simulink library "halout"  (R2021b)
settings: Solver=VariableStepAuto  StartTime=0.0  StopTime=10.0  RelTol=1e-3
undefined symbols (not defined in the file): C_TASK_5MS_S, FALSE, KHAL_CAN1FD1APS3E2E_flg, KHAL_CAN1FD1APS3TxReq_flg, KHAL_CAN1FD1VCU2E2E_flg, KHAL_CAN1FD1VCU2TxReq_flg, KHAL_CAN1FD1VCU3E2E_flg, KHAL_CAN1FD1VCU3TxReq_flg, KHAL_CAN1TxReq_flg, KHAL_CAN1VMCFCM1E2E_flg, KHAL_CAN1VMCFCM1TxReq_flg, KHAL_CAN2TxReq_flg, KHAL_CAN3FD3VCU1toNIDECTxReq_flg, KHAL_CAN3FD3VCU1TxReq_flg, KHAL_CAN3FD3VCU2E2E_flg, KHAL_CAN3FD3VCU2toNIDECE2E_flg, KHAL_CAN3FD3VCU2toNIDECTxReq_flg, KHAL_CAN3FD3VCU2TxReq_flg, KHAL_CAN3TxReq_flg, KHAL_CAN4FD4CE1000E2E_flg, KHAL_CAN4FD4CE1000TxReq_flg, KHAL_CAN4TxReq_flg, KHAL_CAN5TxReq_flg, KHAL_CAN6FD6APS3E2E_flg, KHAL_CAN6FD6APS3TxReq_flg, KHAL_CAN6FD6VCU2E2E_flg, KHAL_CAN6FD6VCU2TxReq_flg, KHAL_CAN6TxReq_flg, ONE_INT, TRUE, ZERO_INT
libraries: FVT_lib x551, simulink x244
(part 16 of 26)

== system halout/HAL_OUT/CAN1/FD1_VCU3_0x159/RrEDURealDrvOrBRgnTq ==
  RrEDURealDrvOrBRgnTq : Inport
  Data Type Conversion : DataTypeConversion  OutDataTypeStr=uint16  RndMeth=Round
  convert_out : FVT_lib/hal/convert_out  gain=0.5  offset=-5300
  CAN1_Rr_EDURealDrvOrBRgnTq : Outport
  wires:
  Data Type Conversion/1 -> CAN1_Rr_EDURealDrvOrBRgnTq/1
  convert_out/1 -> Data Type Conversion/1
  RrEDURealDrvOrBRgnTq/1 -> convert_out/1

== system halout/HAL_OUT/CAN1/FD1_VCU3_0x159/RrEDUSpd ==
  RrEDUSpd : Inport
  Data Type Conversion : DataTypeConversion  OutDataTypeStr=uint16  RndMeth=Round
  convert_out : FVT_lib/hal/convert_out  gain=1  offset=-2000
  CAN1_Rr_EDUSpd : Outport
  wires:
  Data Type Conversion/1 -> CAN1_Rr_EDUSpd/1
  convert_out/1 -> Data Type Conversion/1
  RrEDUSpd/1 -> convert_out/1

== system halout/HAL_OUT/CAN1/FD1_VCU3_0x159/RrEDUSpdValid ==
  RrEDUSpdValid : Inport
  Data Type Conversion : DataTypeConversion  OutDataTypeStr=uint8  RndMeth=Round
  CAN1_Rr_EDUSpdValid : Outport
  wires:
  Data Type Conversion/1 -> CAN1_Rr_EDUSpdValid/1
  RrEDUSpdValid/1 -> Data Type Conversion/1

== system halout/HAL_OUT/CAN1/FD1_VCU3_0x159/RrRgnDecrSta ==
  RrRgnDecrSta : Inport
  Data Type Conversion : DataTypeConversion  OutDataTypeStr=uint8  RndMeth=Round
  CAN1_Rr_RgnDecrSta : Outport
  wires:
  Data Type Conversion/1 -> CAN1_Rr_RgnDecrSta/1
  RrRgnDecrSta/1 -> Data Type Conversion/1

== system halout/HAL_OUT/CAN1/FD1_VCU3_0x159/RrRgnPermSta ==
  RrRgnPermSta : Inport
  Data Type Conversion : DataTypeConversion  OutDataTypeStr=uint8  RndMeth=Round
  CAN1_Rr_RgnPermSta : Outport
  wires:
  Data Type Conversion/1 -> CAN1_Rr_RgnPermSta/1
  RrRgnPermSta/1 -> Data Type Conversion/1

== system halout/HAL_OUT/CAN1/FD1_VMC1_0x17F/AccCalcuPID ==
  AccCalcuPID : Inport
  Data Type Conversion : DataTypeConversion  OutDataTypeStr=uint16  RndMeth=Round
  convert_out : FVT_lib/hal/convert_out  gain=0.05  offset=-15
  CAN1_AccCalcuPID : Outport
  wires:
  Data Type Conversion/1 -> CAN1_AccCalcuPID/1
  convert_out/1 -> Data Type Conversion/1
  AccCalcuPID/1 -> convert_out/1

== system halout/HAL_OUT/CAN1/FD1_VMC1_0x17F/CCMSASpdWar ==
  CCMSASpdWar : Inport
  Data Type Conversion : DataTypeConversion  OutDataTypeStr=uint8  RndMeth=Round
  CAN1_CCMSA_SpdWar : Outport
  wires:
  Data Type Conversion/1 -> CAN1_CCMSA_SpdWar/1
  CCMSASpdWar/1 -> Data Type Conversion/1

== system halout/HAL_OUT/CAN1/FD1_VMC1_0x17F/DISCButtSta ==
  DISCButtSta : Inport
  Data Type Conversion : DataTypeConversion  OutDataTypeStr=uint8  RndMeth=Round
  CAN1_DISC_ButtSta : Outport
  wires:
  Data Type Conversion/1 -> CAN1_DISC_ButtSta/1
  DISCButtSta/1 -> Data Type Conversion/1

== system halout/HAL_OUT/CAN1/FD1_VMC1_0x17F/DISCDISCTargetSpd ==
  DISCDISCTargetSpd : Inport
  Data Type Conversion : DataTypeConversion  OutDataTypeStr=uint16  RndMeth=Round
  convert_out : FVT_lib/hal/convert_out  gain=0.125  offset=0
  CAN1_DISC_DISCTargetSpd : Outport
  wires:
  Data Type Conversion/1 -> CAN1_DISC_DISCTargetSpd/1
  convert_out/1 -> Data Type Conversion/1
  DISCDISCTargetSpd/1 -> convert_out/1

== system halout/HAL_OUT/CAN1/FD1_VMC1_0x17F/DISCDISCTurn ==
  DISCDISCTurn : Inport
  Data Type Conversion : DataTypeConversion  OutDataTypeStr=uint8  RndMeth=Round
  CAN1_DISC_DISCTurn : Outport
  wires:
  Data Type Conversion/1 -> CAN1_DISC_DISCTurn/1
  DISCDISCTurn/1 -> Data Type Conversion/1

== system halout/HAL_OUT/CAN1/FD1_VMC1_0x17F/DISCReqAcc ==
  DISCReqAcc : Inport
  Data Type Conversion : DataTypeConversion  OutDataTypeStr=uint16  RndMeth=Round
  convert_out : FVT_lib/hal/convert_out  gain=0.05  offset=-15
  CAN1_DISCReqAcc : Outport
  wires:
  Data Type Conversion/1 -> CAN1_DISCReqAcc/1
  convert_out/1 -> Data Type Conversion/1
  DISCReqAcc/1 -> convert_out/1

== system halout/HAL_OUT/CAN1/FD1_VMC1_0x17F/DISCSta ==
  DISCSta : Inport
  Data Type Conversion : DataTypeConversion  OutDataTypeStr=uint8  RndMeth=Round
  CAN1_DISC_Sta : Outport
  wires:
  Data Type Conversion/1 -> CAN1_DISC_Sta/1
  DISCSta/1 -> Data Type Conversion/1

== system halout/HAL_OUT/CAN1/FD1_VMC1_0x17F/FeatArbitrFinal ==
  FeatArbitrFinal : Inport
  Data Type Conversion : DataTypeConversion  OutDataTypeStr=uint8  RndMeth=Round
  CAN1_FeatArbitrFinal : Outport
  wires:
  Data Type Conversion/1 -> CAN1_FeatArbitrFinal/1
  FeatArbitrFinal/1 -> Data Type Conversion/1

== system halout/HAL_OUT/CAN1/FD1_VMC1_0x17F/FeatArbitrSta ==
  FeatArbitrSta : Inport
  Data Type Conversion : DataTypeConversion  OutDataTypeStr=uint8  RndMeth=Round
  CAN1_FeatArbitrSta : Outport
  wires:
  Data Type Conversion/1 -> CAN1_FeatArbitrSta/1
  FeatArbitrSta/1 -> Data Type Conversion/1

== system halout/HAL_OUT/CAN1/FD1_VMC1_0x17F/FeatReqSpd ==
  FeatReqSpd : Inport
  Data Type Conversion : DataTypeConversion  OutDataTypeStr=uint16  RndMeth=Round
  convert_out : FVT_lib/hal/convert_out  gain=0.125  offset=0
  CAN1_FeatReqSpd : Outport
  wires:
  Data Type Conversion/1 -> CAN1_FeatReqSpd/1
  convert_out/1 -> Data Type Conversion/1
  FeatReqSpd/1 -> convert_out/1

== system halout/HAL_OUT/CAN1/FD1_VMC1_0x17F/FeatSetSpdFinalraw32 ==
  FeatSetSpdFinalraw32 : Inport
  Data Type Conversion : DataTypeConversion  OutDataTypeStr=uint8  RndMeth=Round
  CAN1_FeatSetSpdFinal_raw32 : Outport
  wires:
  Data Type Conversion/1 -> CAN1_FeatSetSpdFinal_raw32/1
  FeatSetSpdFinalraw32/1 -> Data Type Conversion/1

== system halout/HAL_OUT/CAN1/FD1_VMC1_0x17F/FrontRearSlipRatioCtrl ==
  FrontRearSlipRatioCtrl : Inport
  Data Type Conversion : DataTypeConversion  OutDataTypeStr=uint8  RndMeth=Round
  CAN1_FrontRearSlipRatioCtrl : Outport
  wires:
  Data Type Conversion/1 -> CAN1_FrontRearSlipRatioCtrl/1
  FrontRearSlipRatioCtrl/1 -> Data Type Conversion/1

== system halout/HAL_OUT/CAN1/FD1_VMC1_0x17F/JerkPCT ==
  JerkPCT : Inport
  Data Type Conversion : DataTypeConversion  OutDataTypeStr=uint8  RndMeth=Round
  CAN1_JerkPCT : Outport
  wires:
  Data Type Conversion/1 -> CAN1_JerkPCT/1
  JerkPCT/1 -> Data Type Conversion/1

== system halout/HAL_OUT/CAN1/FD1_VMC1_0x17F/LatAccCtrl ==
  LatAccCtrl : Inport
  Data Type Conversion : DataTypeConversion  OutDataTypeStr=uint8  RndMeth=Round
  CAN1_LatAccCtrl : Outport
  wires:
  Data Type Conversion/1 -> CAN1_LatAccCtrl/1
  LatAccCtrl/1 -> Data Type Conversion/1

== system halout/HAL_OUT/CAN1/FD1_VMC1_0x17F/LateralCtrl ==
  LateralCtrl : Inport
  Data Type Conversion : DataTypeConversion  OutDataTypeStr=uint8  RndMeth=Round
  CAN1_LateralCtrl : Outport
  wires:
  Data Type Conversion/1 -> CAN1_LateralCtrl/1
  LateralCtrl/1 -> Data Type Conversion/1

== system halout/HAL_OUT/CAN1/FD1_VMC1_0x17F/LimitPCT ==
  LimitPCT : Inport
  Data Type Conversion : DataTypeConversion  OutDataTypeStr=uint8  RndMeth=Round
  CAN1_LimitPCT : Outport
  wires:
  Data Type Conversion/1 -> CAN1_LimitPCT/1
  LimitPCT/1 -> Data Type Conversion/1

== system halout/HAL_OUT/CAN1/FD1_VMC1_0x17F/MeterIndSpeedraw32 ==
  MeterIndSpeedraw32 : Inport
  Data Type Conversion : DataTypeConversion  OutDataTypeStr=uint8  RndMeth=Round
  CAN1_MeterIndSpeed_raw32 : Outport
  wires:
  Data Type Conversion/1 -> CAN1_MeterIndSpeed_raw32/1
  MeterIndSpeedraw32/1 -> Data Type Conversion/1

== system halout/HAL_OUT/CAN1/FD1_VMC1_0x17F/RearWhlSlipRatioCtrl ==
  RearWhlSlipRatioCtrl : Inport
  Data Type Conversion : DataTypeConversion  OutDataTypeStr=uint8  RndMeth=Round
  CAN1_RearWhlSlipRatioCtrl : Outport
  wires:
  Data Type Conversion/1 -> CAN1_RearWhlSlipRatioCtrl/1
  RearWhlSlipRatioCtrl/1 -> Data Type Conversion/1

== system halout/HAL_OUT/CAN1/FD1_VMC1_0x17F/SPD2ACCAct ==
  SPD2ACCAct : Inport
  Data Type Conversion : DataTypeConversion  OutDataTypeStr=uint8  RndMeth=Round
  CAN1_SPD2ACCAct : Outport
  wires:
  Data Type Conversion/1 -> CAN1_SPD2ACCAct/1
  SPD2ACCAct/1 -> Data Type Conversion/1

== system halout/HAL_OUT/CAN1/FD1_VMC1_0x17F/SafetyCtrl ==
  SafetyCtrl : Inport
  Data Type Conversion : DataTypeConversion  OutDataTypeStr=uint8  RndMeth=Round
  CAN1_SafetyCtrl : Outport
  wires:
  Data Type Conversion/1 -> CAN1_SafetyCtrl/1
  SafetyCtrl/1 -> Data Type Conversion/1

== system halout/HAL_OUT/CAN1/FD1_VMC1_0x17F/SingleWhlSlipRatioCtrl ==
  SingleWhlSlipRatioCtrl : Inport
  Data Type Conversion : DataTypeConversion  OutDataTypeStr=uint8  RndMeth=Round
  CAN1_SingleWhlSlipRatioCtrl : Outport
  wires:
  Data Type Conversion/1 -> CAN1_SingleWhlSlipRatioCtrl/1
  SingleWhlSlipRatioCtrl/1 -> Data Type Conversion/1

== system halout/HAL_OUT/CAN1/FD1_VMC1_0x17F/TimeGapCalcu ==
  TimeGapCalcu : Inport
  Data Type Conversion : DataTypeConversion  OutDataTypeStr=uint8  RndMeth=Round
  convert_out : FVT_lib/hal/convert_out  gain=0.1  offset=0
  CAN1_TimeGapCalcu : Outport
  wires:
  Data Type Conversion/1 -> CAN1_TimeGapCalcu/1
  convert_out/1 -> Data Type Conversion/1
  TimeGapCalcu/1 -> convert_out/1

== system halout/HAL_OUT/CAN1/FD1_VMC1_0x17F/VMCACCCtrlAvail ==
  VMCACCCtrlAvail : Inport
  Data Type Conversion : DataTypeConversion  OutDataTypeStr=uint8  RndMeth=Round
  CAN1_VMC_ACCCtrlAvail : Outport
  wires:
  Data Type Conversion/1 -> CAN1_VMC_ACCCtrlAvail/1
  VMCACCCtrlAvail/1 -> Data Type Conversion/1

== system halout/HAL_OUT/CAN1/FD1_VMC1_0x17F/VMCAEBCtrlAvail ==
  VMCAEBCtrlAvail : Inport
  Data Type Conversion : DataTypeConversion  OutDataTypeStr=uint8  RndMeth=Round
  CAN1_VMC_AEBCtrlAvail : Outport
  wires:
  Data Type Conversion/1 -> CAN1_VMC_AEBCtrlAvail/1
  VMCAEBCtrlAvail/1 -> Data Type Conversion/1

== system halout/HAL_OUT/CAN1/FD1_VMC1_0x17F/VMCCCCtrlAvail ==
  VMCCCCtrlAvail : Inport
  Data Type Conversion : DataTypeConversion  OutDataTypeStr=uint8  RndMeth=Round
  CAN1_VMC_CCCtrlAvail : Outport
  wires:
  Data Type Conversion/1 -> CAN1_VMC_CCCtrlAvail/1
  VMCCCCtrlAvail/1 -> Data Type Conversion/1

== system halout/HAL_OUT/CAN1/FD1_VMC1_0x17F/VMCMSACtrlAvail ==
  VMCMSACtrlAvail : Inport
  Data Type Conversion : DataTypeConversion  OutDataTypeStr=uint8  RndMeth=Round
  CAN1_VMC_MSACtrlAvail : Outport
  wires:
  Data Type Conversion/1 -> CAN1_VMC_MSACtrlAvail/1
  VMCMSACtrlAvail/1 -> Data Type Conversion/1

== system halout/HAL_OUT/CAN1/FD1_VMC1_0x17F/VMCVCUACCCtrlAvail ==
  VMCVCUACCCtrlAvail : Inport
  Data Type Conversion : DataTypeConversion  OutDataTypeStr=uint8  RndMeth=Round
  CAN1_VMC_VCU_ACC_CtrlAvail : Outport
  wires:
  Data Type Conversion/1 -> CAN1_VMC_VCU_ACC_CtrlAvail/1
  VMCVCUACCCtrlAvail/1 -> Data Type Conversion/1

== system halout/HAL_OUT/CAN1/FD1_VMC1_0x17F/VMCVCUAPSCtrlAvailflg ==
  VMCVCUAPSCtrlAvailflg : Inport
  Data Type Conversion : DataTypeConversion  OutDataTypeStr=uint8  RndMeth=Round
  CAN1_VMC_VCU_APSCtrlAvail_flg : Outport
  wires:
  Data Type Conversion/1 -> CAN1_VMC_VCU_APSCtrlAvail_flg/1
  VMCVCUAPSCtrlAvailflg/1 -> Data Type Conversion/1

== system halout/HAL_OUT/CAN1/FD1_VMC1_0x17F/VMCVCUAccPedalOverride ==
  VMCVCUAccPedalOverride : Inport
  Data Type Conversion : DataTypeConversion  OutDataTypeStr=uint8  RndMeth=Round
  CAN1_VMC_VCU_AccPedal_Override : Outport
  wires:
  Data Type Conversion/1 -> CAN1_VMC_VCU_AccPedal_Override/1
  VMCVCUAccPedalOverride/1 -> Data Type Conversion/1

== system halout/HAL_OUT/CAN1/FD1_VMC1_0x17F/VMCVCUCCCrlSta ==
  VMCVCUCCCrlSta : Inport
  Data Type Conversion : DataTypeConversion  OutDataTypeStr=uint8  RndMeth=Round
  CAN1_VMC_VCU_CC_Crl_Sta : Outport
  wires:
  Data Type Conversion/1 -> CAN1_VMC_VCU_CC_Crl_Sta/1
  VMCVCUCCCrlSta/1 -> Data Type Conversion/1

== system halout/HAL_OUT/CAN1/FD1_VMC1_0x17F/VMCVCUMSACrlSta ==
  VMCVCUMSACrlSta : Inport
  Data Type Conversion : DataTypeConversion  OutDataTypeStr=uint8  RndMeth=Round
  CAN1_VMC_VCU_MSA_Crl_Sta : Outport
  wires:
  Data Type Conversion/1 -> CAN1_VMC_VCU_MSA_Crl_Sta/1
  VMCVCUMSACrlSta/1 -> Data Type Conversion/1

== system halout/HAL_OUT/CAN1/FD1_VMC1_0x17F/VehicleSpeedkph ==
  VehicleSpeedkph : Inport
  Data Type Conversion : DataTypeConversion  OutDataTypeStr=uint16  RndMeth=Round
  convert_out : FVT_lib/hal/convert_out  gain=0.125  offset=0
  CAN1_VehicleSpeed_kph : Outport
  wires:
  Data Type Conversion/1 -> CAN1_VehicleSpeed_kph/1
  convert_out/1 -> Data Type Conversion/1
  VehicleSpeedkph/1 -> convert_out/1

== system halout/HAL_OUT/CAN1/FD1_VMC1_0x17F/VehicleSpeedmph ==
  VehicleSpeedmph : Inport
  Data Type Conversion : DataTypeConversion  OutDataTypeStr=uint16  RndMeth=Round
  convert_out : FVT_lib/hal/convert_out  gain=0.125  offset=0
  CAN1_VehicleSpeed_mph : Outport
  wires:
  Data Type Conversion/1 -> CAN1_VehicleSpeed_mph/1
  convert_out/1 -> Data Type Conversion/1
  VehicleSpeedmph/1 -> convert_out/1

== system halout/HAL_OUT/CAN1/FD1_VMC2_0x77/FDCVMCRWSActvSta ==
  FDCVMCRWSActvSta : Inport
  Data Type Conversion : DataTypeConversion  OutDataTypeStr=uint8  RndMeth=Round
  CAN1_FDC_VMC_RWS_Actv_Sta : Outport
  wires:
  Data Type Conversion/1 -> CAN1_FDC_VMC_RWS_Actv_Sta/1
  FDCVMCRWSActvSta/1 -> Data Type Conversion/1

== system halout/HAL_OUT/CAN1/FD1_VMC2_0x77/FDCVMCRWSDfctvSta ==
  FDCVMCRWSDfctvSta : Inport
  Data Type Conversion : DataTypeConversion  OutDataTypeStr=uint8  RndMeth=Round
  CAN1_FDC_VMC_RWS_Dfctv_Sta : Outport
  wires:
  Data Type Conversion/1 -> CAN1_FDC_VMC_RWS_Dfctv_Sta/1
  FDCVMCRWSDfctvSta/1 -> Data Type Conversion/1

== system halout/HAL_OUT/CAN1/FD1_VMC2_0x77/FDCVMCRWSPositionReqCmd ==
  FDCVMCRWSPositionReqCmd : Inport
  Data Type Conversion : DataTypeConversion  OutDataTypeStr=uint16  RndMeth=Round
  convert_out : FVT_lib/hal/convert_out  gain=0.01  offset=-327.67
  CAN1_FDC_VMC_RWS_PositionReq_Cmd : Outport
  wires:
  Data Type Conversion/1 -> CAN1_FDC_VMC_RWS_PositionReq_Cmd/1
  convert_out/1 -> Data Type Conversion/1
  FDCVMCRWSPositionReqCmd/1 -> convert_out/1

== system halout/HAL_OUT/CAN1/FD1_VMC2_0x77/FDCVMCSteerFaultReqCmd ==
  FDCVMCSteerFaultReqCmd : Inport
  Data Type Conversion : DataTypeConversion  OutDataTypeStr=uint8  RndMeth=Round
  CAN1_FDC_VMC_SteerFaultReq_Cmd : Outport
  wires:
  Data Type Conversion/1 -> CAN1_FDC_VMC_SteerFaultReq_Cmd/1
  FDCVMCSteerFaultReqCmd/1 -> Data Type Conversion/1

== system halout/HAL_OUT/CAN1/VMC_FCM1_0x172/Byte_0 ==
  VMC_FCM1_Checksum : Inport
  BitwiseOR : simulink/Logic and Bit Operations/Bitwise Operator  logicop=OR  UseBitMask=off  BitMask=bin2dec('11011001')  BitMaskRealWorld=Stored Integer
  SignalPack : FVT_lib/hal/SignalPack  RightShiftCnt=0  BitMask=2^8-1  LeftShiftCnt=0
  UnitConverter : DataTypeConversion  OutDataTypeStr=uint8  RndMeth=Round
  UnitConverter1 : DataTypeConversion  OutDataTypeStr=uint8  RndMeth=Round
  Byte_0 : Outport
  wires:
  BitwiseOR/1 -> Byte_0/1
  UnitConverter/1 -> BitwiseOR/1
  SignalPack/1 -> UnitConverter/1
  UnitConverter1/1 -> SignalPack/1
  VMC_FCM1_Checksum/1 -> UnitConverter1/1

== system halout/HAL_OUT/CAN1/VMC_FCM1_0x172/Byte_1 ==
  VMC_FCM1_LifeCount : Inport
  BitwiseOR : simulink/Logic and Bit Operations/Bitwise Operator  logicop=OR  UseBitMask=off  BitMask=bin2dec('11011001')  BitMaskRealWorld=Stored Integer
  SignalPack : FVT_lib/hal/SignalPack  RightShiftCnt=0  BitMask=2^4-1  LeftShiftCnt=0
  UnitConverter : DataTypeConversion  OutDataTypeStr=uint8  RndMeth=Round
  UnitConverter1 : DataTypeConversion  OutDataTypeStr=uint8  RndMeth=Round
  Byte_1 : Outport
  wires:
  BitwiseOR/1 -> Byte_1/1
  UnitConverter/1 -> BitwiseOR/1
  SignalPack/1 -> UnitConverter/1
  UnitConverter1/1 -> SignalPack/1
  VMC_FCM1_LifeCount/1 -> UnitConverter1/1

== system halout/HAL_OUT/CAN1/VMC_FCM1_0x172/Byte_10 ==
  VMC_ACC_ComfortBandLower : Inport
  BitwiseOR : simulink/Logic and Bit Operations/Bitwise Operator  logicop=OR  UseBitMask=off  BitMask=bin2dec('11011001')  BitMaskRealWorld=Stored Integer
  SignalPack : FVT_lib/hal/SignalPack  RightShiftCnt=0  BitMask=2^8-1  LeftShiftCnt=0
  UnitConverter : DataTypeConversion  OutDataTypeStr=uint8  RndMeth=Round
  UnitConverter1 : DataTypeConversion  OutDataTypeStr=uint16  RndMeth=Round
  convert_out : FVT_lib/hal/convert_out  gain=0.05  offset=-15
  Byte_10 : Outport
  wires:
  BitwiseOR/1 -> Byte_10/1
  UnitConverter/1 -> BitwiseOR/1
  SignalPack/1 -> UnitConverter/1
  UnitConverter1/1 -> SignalPack/1
  convert_out/1 -> UnitConverter1/1
  VMC_ACC_ComfortBandLower/1 -> convert_out/1

== system halout/HAL_OUT/CAN1/VMC_FCM1_0x172/Byte_11 ==
  FDC_VMC_DrInpTqBstAct : Inport
  FDC_VMC_MaxAngCtrlOutTqLim : Inport  Port=2
  VMC_ADAS_ACC_Sta : Inport  Port=3
  VMC_ADAS_AEB_Sta : Inport  Port=4
  BitwiseOR : simulink/Logic and Bit Operations/Bitwise Operator  logicop=OR  UseBitMask=off  NumInputPorts=4  BitMask=bin2dec('11011001')  BitMaskRealWorld=Stored Integer
  SignalPack : FVT_lib/hal/SignalPack  RightShiftCnt=0  BitMask=2^1-1  LeftShiftCnt=1
  SignalPack1 : FVT_lib/hal/SignalPack  RightShiftCnt=8  BitMask=2^1-1  LeftShiftCnt=0
  SignalPack2 : FVT_lib/hal/SignalPack  RightShiftCnt=0  BitMask=2^3-1  LeftShiftCnt=5
  SignalPack3 : FVT_lib/hal/SignalPack  RightShiftCnt=0  BitMask=2^3-1  LeftShiftCnt=2
  UnitConverter{,1..2,4..7} (7 alike) : DataTypeConversion  OutDataTypeStr=uint8  RndMeth=Round
  UnitConverter3 : DataTypeConversion  OutDataTypeStr=uint16  RndMeth=Round
  convert_out : FVT_lib/hal/convert_out  gain=0.1  offset=0
  Byte_11 : Outport
  wires:
  BitwiseOR/1 -> Byte_11/1
  UnitConverter/1 -> BitwiseOR/1
  SignalPack/1 -> UnitConverter/1
  UnitConverter1/1 -> SignalPack/1
  FDC_VMC_DrInpTqBstAct/1 -> UnitConverter1/1
  UnitConverter2/1 -> BitwiseOR/2
  SignalPack1/1 -> UnitConverter2/1
  UnitConverter3/1 -> SignalPack1/1
  convert_out/1 -> UnitConverter3/1
  FDC_VMC_MaxAngCtrlOutTqLim/1 -> convert_out/1
  UnitConverter4/1 -> BitwiseOR/3
  SignalPack2/1 -> UnitConverter4/1
  UnitConverter5/1 -> SignalPack2/1
  VMC_ADAS_ACC_Sta/1 -> UnitConverter5/1
  UnitConverter6/1 -> BitwiseOR/4
  SignalPack3/1 -> UnitConverter6/1
  UnitConverter7/1 -> SignalPack3/1
  VMC_ADAS_AEB_Sta/1 -> UnitConverter7/1

== system halout/HAL_OUT/CAN1/VMC_FCM1_0x172/Byte_12 ==
  FDC_VMC_MaxAngCtrlOutTqLim : Inport
  BitwiseOR : simulink/Logic and Bit Operations/Bitwise Operator  logicop=OR  UseBitMask=off  BitMask=bin2dec('11011001')  BitMaskRealWorld=Stored Integer
  SignalPack : FVT_lib/hal/SignalPack  RightShiftCnt=0  BitMask=2^8-1  LeftShiftCnt=0
  UnitConverter : DataTypeConversion  OutDataTypeStr=uint8  RndMeth=Round
  UnitConverter1 : DataTypeConversion  OutDataTypeStr=uint16  RndMeth=Round
  convert_out : FVT_lib/hal/convert_out  gain=0.1  offset=0
  Byte_12 : Outport
  wires:
  BitwiseOR/1 -> Byte_12/1
  UnitConverter/1 -> BitwiseOR/1
  SignalPack/1 -> UnitConverter/1
  UnitConverter1/1 -> SignalPack/1
  convert_out/1 -> UnitConverter1/1
  FDC_VMC_MaxAngCtrlOutTqLim/1 -> convert_out/1

== system halout/HAL_OUT/CAN1/VMC_FCM1_0x172/Byte_13 ==
  FDC_VMC_AngCtrlTqWtGn : Inport
  BitwiseOR : simulink/Logic and Bit Operations/Bitwise Operator  logicop=OR  UseBitMask=off  BitMask=bin2dec('11011001')  BitMaskRealWorld=Stored Integer
  SignalPack : FVT_lib/hal/SignalPack  RightShiftCnt=0  BitMask=2^8-1  LeftShiftCnt=0
  UnitConverter : DataTypeConversion  OutDataTypeStr=uint8  RndMeth=Round
  UnitConverter1 : DataTypeConversion  OutDataTypeStr=uint8  RndMeth=Round
  convert_out : FVT_lib/hal/convert_out  gain=0.4  offset=0
  Byte_13 : Outport
  wires:
  BitwiseOR/1 -> Byte_13/1
  UnitConverter/1 -> BitwiseOR/1
  SignalPack/1 -> UnitConverter/1
  UnitConverter1/1 -> SignalPack/1
  convert_out/1 -> UnitConverter1/1
  FDC_VMC_AngCtrlTqWtGn/1 -> convert_out/1

== system halout/HAL_OUT/CAN1/VMC_FCM1_0x172/Byte_14 ==
  FDC_VMC_DrInpTqBstGn : Inport
  BitwiseOR : simulink/Logic and Bit Operations/Bitwise Operator  logicop=OR  UseBitMask=off  BitMask=bin2dec('11011001')  BitMaskRealWorld=Stored Integer
  SignalPack : FVT_lib/hal/SignalPack  RightShiftCnt=0  BitMask=2^8-1  LeftShiftCnt=0
  UnitConverter : DataTypeConversion  OutDataTypeStr=uint8  RndMeth=Round
  UnitConverter1 : DataTypeConversion  OutDataTypeStr=uint8  RndMeth=Round
  convert_out : FVT_lib/hal/convert_out  gain=0.4  offset=0
  Byte_14 : Outport
  wires:
  BitwiseOR/1 -> Byte_14/1
  UnitConverter/1 -> BitwiseOR/1
  SignalPack/1 -> UnitConverter/1
  UnitConverter1/1 -> SignalPack/1
  convert_out/1 -> UnitConverter1/1
  FDC_VMC_DrInpTqBstGn/1 -> convert_out/1

== system halout/HAL_OUT/CAN1/VMC_FCM1_0x172/Byte_15 ==
  FDC_VMC_DMSMode_Cmd : Inport
  BitwiseOR : simulink/Logic and Bit Operations/Bitwise Operator  logicop=OR  UseBitMask=off  BitMask=bin2dec('11011001')  BitMaskRealWorld=Stored Integer
  SignalPack : FVT_lib/hal/SignalPack  RightShiftCnt=0  BitMask=2^4-1  LeftShiftCnt=0
  UnitConverter : DataTypeConversion  OutDataTypeStr=uint8  RndMeth=Round
  UnitConverter1 : DataTypeConversion  OutDataTypeStr=uint8  RndMeth=Round
  Byte_15 : Outport
  wires:
  BitwiseOR/1 -> Byte_15/1
  UnitConverter/1 -> BitwiseOR/1
  SignalPack/1 -> UnitConverter/1
  UnitConverter1/1 -> SignalPack/1
  FDC_VMC_DMSMode_Cmd/1 -> UnitConverter1/1

== system halout/HAL_OUT/CAN1/VMC_FCM1_0x172/Byte_2 ==
  VMC_FCM_LKA_TOIAct : Inport
  BitwiseOR : simulink/Logic and Bit Operations/Bitwise Operator  logicop=OR  UseBitMask=off  BitMask=bin2dec('11011001')  BitMaskRealWorld=Stored Integer
  SignalPack : FVT_lib/hal/SignalPack  RightShiftCnt=0  BitMask=2^8-1  LeftShiftCnt=0
  UnitConverter : DataTypeConversion  OutDataTypeStr=uint8  RndMeth=Round
  UnitConverter1 : DataTypeConversion  OutDataTypeStr=uint8  RndMeth=Round
  Byte_2 : Outport
  wires:
  BitwiseOR/1 -> Byte_2/1
  UnitConverter/1 -> BitwiseOR/1
  SignalPack/1 -> UnitConverter/1
  UnitConverter1/1 -> SignalPack/1
  VMC_FCM_LKA_TOIAct/1 -> UnitConverter1/1

== system halout/HAL_OUT/CAN1/VMC_FCM1_0x172/Byte_3 ==
  VMC_AEB_VehHoldReq : Inport
  VMC_FCM_LDW_Fault : Inport  Port=2
  VMC_FCM_LDW_Request : Inport  Port=3
  VMC_FCM_LKA_StrToqReq : Inport  Port=4
  VMC_FCM_LKA_TOIFault : Inport  Port=5
  BitwiseOR : simulink/Logic and Bit Operations/Bitwise Operator  logicop=OR  UseBitMask=off  NumInputPorts=5  BitMask=bin2dec('11011001')  BitMaskRealWorld=Stored Integer
  SignalPack : FVT_lib/hal/SignalPack  RightShiftCnt=0  BitMask=2^1-1  LeftShiftCnt=3
  SignalPack1 : FVT_lib/hal/SignalPack  RightShiftCnt=0  BitMask=2^1-1  LeftShiftCnt=5
  SignalPack2 : FVT_lib/hal/SignalPack  RightShiftCnt=0  BitMask=2^2-1  LeftShiftCnt=6
  SignalPack3 : FVT_lib/hal/SignalPack  RightShiftCnt=8  BitMask=2^3-1  LeftShiftCnt=0
  SignalPack4 : FVT_lib/hal/SignalPack  RightShiftCnt=0  BitMask=2^1-1  LeftShiftCnt=4
  UnitConverter{,1..6,8..9} (9 alike) : DataTypeConversion  OutDataTypeStr=uint8  RndMeth=Round
  UnitConverter7 : DataTypeConversion  OutDataTypeStr=uint16  RndMeth=Round
  convert_out : FVT_lib/hal/convert_out  gain=0.008  offset=-8
  Byte_3 : Outport
  wires:
  BitwiseOR/1 -> Byte_3/1
  UnitConverter/1 -> BitwiseOR/1
  SignalPack/1 -> UnitConverter/1
  UnitConverter1/1 -> SignalPack/1
  VMC_AEB_VehHoldReq/1 -> UnitConverter1/1
  UnitConverter2/1 -> BitwiseOR/2
  SignalPack1/1 -> UnitConverter2/1
  UnitConverter3/1 -> SignalPack1/1
  VMC_FCM_LDW_Fault/1 -> UnitConverter3/1
  UnitConverter4/1 -> BitwiseOR/3
  SignalPack2/1 -> UnitConverter4/1
  UnitConverter5/1 -> SignalPack2/1
  VMC_FCM_LDW_Request/1 -> UnitConverter5/1
  UnitConverter6/1 -> BitwiseOR/4
  SignalPack3/1 -> UnitConverter6/1
  UnitConverter7/1 -> SignalPack3/1
  convert_out/1 -> UnitConverter7/1
  VMC_FCM_LKA_StrToqReq/1 -> convert_out/1
  UnitConverter8/1 -> BitwiseOR/5
  SignalPack4/1 -> UnitConverter8/1
  UnitConverter9/1 -> SignalPack4/1
  VMC_FCM_LKA_TOIFault/1 -> UnitConverter9/1

== system halout/HAL_OUT/CAN1/VMC_FCM1_0x172/Byte_4 ==
  VMC_FCM_LKA_StrToqReq : Inport
  BitwiseOR : simulink/Logic and Bit Operations/Bitwise Operator  logicop=OR  UseBitMask=off  BitMask=bin2dec('11011001')  BitMaskRealWorld=Stored Integer
  SignalPack : FVT_lib/hal/SignalPack  RightShiftCnt=0  BitMask=2^8-1  LeftShiftCnt=0
  UnitConverter : DataTypeConversion  OutDataTypeStr=uint8  RndMeth=Round
  UnitConverter1 : DataTypeConversion  OutDataTypeStr=uint16  RndMeth=Round
  convert_out : FVT_lib/hal/convert_out  gain=0.008  offset=-8
  Byte_4 : Outport
  wires:
  BitwiseOR/1 -> Byte_4/1
  UnitConverter/1 -> BitwiseOR/1
  SignalPack/1 -> UnitConverter/1
  UnitConverter1/1 -> SignalPack/1
  convert_out/1 -> UnitConverter1/1
  VMC_FCM_LKA_StrToqReq/1 -> convert_out/1

== system halout/HAL_OUT/CAN1/VMC_FCM1_0x172/Byte_5 ==
  VMC_ACC_RequiredAccel : Inport
  VMC_ACC_VehHoldReq : Inport  Port=2
  VMC_ADAS_AEBReq : Inport  Port=3
  VMC_ADAS_DBSReq : Inport  Port=4
  VMC_ADAS_FaultSta : Inport  Port=5
  BitwiseOR : simulink/Logic and Bit Operations/Bitwise Operator  logicop=OR  UseBitMask=off  NumInputPorts=5  BitMask=bin2dec('11011001')  BitMaskRealWorld=Stored Integer
  SignalPack : FVT_lib/hal/SignalPack  RightShiftCnt=8  BitMask=2^1-1  LeftShiftCnt=0
  SignalPack1 : FVT_lib/hal/SignalPack  RightShiftCnt=0  BitMask=2^1-1  LeftShiftCnt=7
  SignalPack2 : FVT_lib/hal/SignalPack  RightShiftCnt=0  BitMask=2^3-1  LeftShiftCnt=1
  SignalPack3 : FVT_lib/hal/SignalPack  RightShiftCnt=0  BitMask=2^2-1  LeftShiftCnt=5
  SignalPack4 : FVT_lib/hal/SignalPack  RightShiftCnt=0  BitMask=2^1-1  LeftShiftCnt=4
  UnitConverter{,2..9} (9 alike) : DataTypeConversion  OutDataTypeStr=uint8  RndMeth=Round
  UnitConverter1 : DataTypeConversion  OutDataTypeStr=uint16  RndMeth=Round
  convert_out : FVT_lib/hal/convert_out  gain=0.05  offset=-15
  Byte_5 : Outport
  wires:
  BitwiseOR/1 -> Byte_5/1
  UnitConverter/1 -> BitwiseOR/1
  SignalPack/1 -> UnitConverter/1
  UnitConverter1/1 -> SignalPack/1
  convert_out/1 -> UnitConverter1/1
  VMC_ACC_RequiredAccel/1 -> convert_out/1
  UnitConverter2/1 -> BitwiseOR/2
  SignalPack1/1 -> UnitConverter2/1
  UnitConverter3/1 -> SignalPack1/1
  VMC_ACC_VehHoldReq/1 -> UnitConverter3/1
  UnitConverter4/1 -> BitwiseOR/3
  SignalPack2/1 -> UnitConverter4/1
  UnitConverter5/1 -> SignalPack2/1
  VMC_ADAS_AEBReq/1 -> UnitConverter5/1
  UnitConverter6/1 -> BitwiseOR/4
  SignalPack3/1 -> UnitConverter6/1
  UnitConverter7/1 -> SignalPack3/1
  VMC_ADAS_DBSReq/1 -> UnitConverter7/1
  UnitConverter8/1 -> BitwiseOR/5
  SignalPack4/1 -> UnitConverter8/1
  UnitConverter9/1 -> SignalPack4/1
  VMC_ADAS_FaultSta/1 -> UnitConverter9/1

== system halout/HAL_OUT/CAN1/VMC_FCM1_0x172/Byte_6 ==
  VMC_ACC_RequiredAccel : Inport
  BitwiseOR : simulink/Logic and Bit Operations/Bitwise Operator  logicop=OR  UseBitMask=off  BitMask=bin2dec('11011001')  BitMaskRealWorld=Stored Integer
  SignalPack : FVT_lib/hal/SignalPack  RightShiftCnt=0  BitMask=2^8-1  LeftShiftCnt=0
  UnitConverter : DataTypeConversion  OutDataTypeStr=uint8  RndMeth=Round
  UnitConverter1 : DataTypeConversion  OutDataTypeStr=uint16  RndMeth=Round
  convert_out : FVT_lib/hal/convert_out  gain=0.05  offset=-15
  Byte_6 : Outport
  wires:
  BitwiseOR/1 -> Byte_6/1
  UnitConverter/1 -> BitwiseOR/1
  SignalPack/1 -> UnitConverter/1
  UnitConverter1/1 -> SignalPack/1
  convert_out/1 -> UnitConverter1/1
  VMC_ACC_RequiredAccel/1 -> convert_out/1

== system halout/HAL_OUT/CAN1/VMC_FCM1_0x172/Byte_7 ==
  VMC_ACC_ComfortBandUpper : Inport
  VMC_ACC_JerkUpperLInit : Inport  Port=2
  BitwiseOR : simulink/Logic and Bit Operations/Bitwise Operator  logicop=OR  UseBitMask=off  NumInputPorts=2  BitMask=bin2dec('11011001')  BitMaskRealWorld=Stored Integer
  SignalPack : FVT_lib/hal/SignalPack  RightShiftCnt=8  BitMask=2^1-1  LeftShiftCnt=0
  SignalPack1 : FVT_lib/hal/SignalPack  RightShiftCnt=0  BitMask=2^7-1  LeftShiftCnt=1
  UnitConverter : DataTypeConversion  OutDataTypeStr=uint8  RndMeth=Round
  UnitConverter1 : DataTypeConversion  OutDataTypeStr=uint16  RndMeth=Round
  UnitConverter2 : DataTypeConversion  OutDataTypeStr=uint8  RndMeth=Round
  UnitConverter3 : DataTypeConversion  OutDataTypeStr=uint8  RndMeth=Round
  convert_out : FVT_lib/hal/convert_out  gain=0.05  offset=-15
  convert_out1 : FVT_lib/hal/convert_out  gain=0.1  offset=-6
  Byte_7 : Outport
  wires:
  BitwiseOR/1 -> Byte_7/1
  UnitConverter/1 -> BitwiseOR/1
  SignalPack/1 -> UnitConverter/1
  UnitConverter1/1 -> SignalPack/1
  convert_out/1 -> UnitConverter1/1
  VMC_ACC_ComfortBandUpper/1 -> convert_out/1
  UnitConverter2/1 -> BitwiseOR/2
  SignalPack1/1 -> UnitConverter2/1
  UnitConverter3/1 -> SignalPack1/1
  convert_out1/1 -> UnitConverter3/1
  VMC_ACC_JerkUpperLInit/1 -> convert_out1/1

== system halout/HAL_OUT/CAN1/VMC_FCM1_0x172/Byte_8 ==
  VMC_ACC_ComfortBandUpper : Inport
  BitwiseOR : simulink/Logic and Bit Operations/Bitwise Operator  logicop=OR  UseBitMask=off  BitMask=bin2dec('11011001')  BitMaskRealWorld=Stored Integer
  SignalPack : FVT_lib/hal/SignalPack  RightShiftCnt=0  BitMask=2^8-1  LeftShiftCnt=0
  UnitConverter : DataTypeConversion  OutDataTypeStr=uint8  RndMeth=Round
  UnitConverter1 : DataTypeConversion  OutDataTypeStr=uint16  RndMeth=Round
  convert_out : FVT_lib/hal/convert_out  gain=0.05  offset=-15
  Byte_8 : Outport
  wires:
  BitwiseOR/1 -> Byte_8/1
  UnitConverter/1 -> BitwiseOR/1
  SignalPack/1 -> UnitConverter/1
  UnitConverter1/1 -> SignalPack/1
  convert_out/1 -> UnitConverter1/1
  VMC_ACC_ComfortBandUpper/1 -> convert_out/1

== system halout/HAL_OUT/CAN1/VMC_FCM1_0x172/Byte_9 ==
  VMC_ACC_ComfortBandLower : Inport
  VMC_ACC_JerkLowerLInit : Inport  Port=2
  BitwiseOR : simulink/Logic and Bit Operations/Bitwise Operator  logicop=OR  UseBitMask=off  NumInputPorts=2  BitMask=bin2dec('11011001')  BitMaskRealWorld=Stored Integer
  SignalPack : FVT_lib/hal/SignalPack  RightShiftCnt=8  BitMask=2^1-1  LeftShiftCnt=0
  SignalPack1 : FVT_lib/hal/SignalPack  RightShiftCnt=0  BitMask=2^7-1  LeftShiftCnt=1
  UnitConverter : DataTypeConversion  OutDataTypeStr=uint8  RndMeth=Round
  UnitConverter1 : DataTypeConversion  OutDataTypeStr=uint16  RndMeth=Round
  UnitConverter2 : DataTypeConversion  OutDataTypeStr=uint8  RndMeth=Round
  UnitConverter3 : DataTypeConversion  OutDataTypeStr=uint8  RndMeth=Round
  convert_out : FVT_lib/hal/convert_out  gain=0.05  offset=-15
  convert_out1 : FVT_lib/hal/convert_out  gain=0.1  offset=-6
  Byte_9 : Outport
  wires:
  BitwiseOR/1 -> Byte_9/1
  UnitConverter/1 -> BitwiseOR/1
  SignalPack/1 -> UnitConverter/1
  UnitConverter1/1 -> SignalPack/1
  convert_out/1 -> UnitConverter1/1
  VMC_ACC_ComfortBandLower/1 -> convert_out/1
  UnitConverter2/1 -> BitwiseOR/2
  SignalPack1/1 -> UnitConverter2/1
  UnitConverter3/1 -> SignalPack1/1
  convert_out1/1 -> UnitConverter3/1
  VMC_ACC_JerkLowerLInit/1 -> convert_out1/1

== system halout/HAL_OUT/CAN1/VMC_FCM1_0x172/CRC8_IfAction_Tx ==
  CAN_E2E_flg : Inport
  DataID1 : Inport  Port=2
  DataID2 : Inport  Port=3
  RawData : Inport  Port=4
  Data Type Conversion : DataTypeConversion  OutDataTypeStr=uint8
  If : If
  If Action Subsystem : Subsystem  TreatAsAtomicUnit=on
  If Action Subsystem1 : Subsystem  TreatAsAtomicUnit=on
  Merge : Merge
  CRC8 : Outport
  wires:
  If/2 -> If Action Subsystem/Action
  If/1 -> If Action Subsystem1/Action
  CAN_E2E_flg/1 -> [CAN_E2E_flg]
  DataID1/1 -> [DataID1]
  DataID2/1 -> [DataID2]
  RawData/1 -> [RawData]
  [CAN_E2E_flg] -> Data Type Conversion/1
  [DataID1] -> If Action Subsystem1/1(CAN_E2E_ID1)
  [DataID2] -> If Action Subsystem1/2(CAN_E2E_ID2)
  [RawData] -> If Action Subsystem1/3(Byte1)
  [RawData] -> If Action Subsystem/1(Byte1)
  If Action Subsystem1/1(CRC8_E2EResult) -> Merge/1
  If Action Subsystem/1(CRC8_Result) -> Merge/2
  Merge/1 -> CRC8/1
  Data Type Conversion/1 -> If/1

== system halout/HAL_OUT/CAN1/VMC_FCM1_0x172/FDCVMCAngCtrlTqWtGn ==
  FDCVMCAngCtrlTqWtGn : Inport
  Data Type Conversion : DataTypeConversion  OutDataTypeStr=uint8  RndMeth=Round
  convert_out : FVT_lib/hal/convert_out  gain=0.4  offset=0
  CAN1_FDC_VMC_AngCtrlTqWtGn : Outport
  wires:
  Data Type Conversion/1 -> CAN1_FDC_VMC_AngCtrlTqWtGn/1
  convert_out/1 -> Data Type Conversion/1
  FDCVMCAngCtrlTqWtGn/1 -> convert_out/1

== system halout/HAL_OUT/CAN1/VMC_FCM1_0x172/FDCVMCDMSModeCmd ==
  FDCVMCDMSModeCmd : Inport
  Data Type Conversion : DataTypeConversion  OutDataTypeStr=uint8  RndMeth=Round
  CAN1_FDC_VMC_DMSMode_Cmd : Outport
  wires:
  Data Type Conversion/1 -> CAN1_FDC_VMC_DMSMode_Cmd/1
  FDCVMCDMSModeCmd/1 -> Data Type Conversion/1

== system halout/HAL_OUT/CAN1/VMC_FCM1_0x172/FDCVMCDrInpTqBstAct ==
  FDCVMCDrInpTqBstAct : Inport
  Data Type Conversion : DataTypeConversion  OutDataTypeStr=uint8  RndMeth=Round
  CAN1_FDC_VMC_DrInpTqBstAct : Outport
  wires:
  Data Type Conversion/1 -> CAN1_FDC_VMC_DrInpTqBstAct/1
  FDCVMCDrInpTqBstAct/1 -> Data Type Conversion/1

== system halout/HAL_OUT/CAN1/VMC_FCM1_0x172/FDCVMCDrInpTqBstGn ==
  FDCVMCDrInpTqBstGn : Inport
  Data Type Conversion : DataTypeConversion  OutDataTypeStr=uint8  RndMeth=Round
  convert_out : FVT_lib/hal/convert_out  gain=0.4  offset=0
  CAN1_FDC_VMC_DrInpTqBstGn : Outport
  wires:
  Data Type Conversion/1 -> CAN1_FDC_VMC_DrInpTqBstGn/1
  convert_out/1 -> Data Type Conversion/1
  FDCVMCDrInpTqBstGn/1 -> convert_out/1

== system halout/HAL_OUT/CAN1/VMC_FCM1_0x172/FDCVMCMaxAngCtrlOutTqLim ==
  FDCVMCMaxAngCtrlOutTqLim : Inport
  Data Type Conversion : DataTypeConversion  OutDataTypeStr=uint16  RndMeth=Round
  convert_out : FVT_lib/hal/convert_out  gain=0.1  offset=0
  CAN1_FDC_VMC_MaxAngCtrlOutTqLim : Outport
  wires:
  Data Type Conversion/1 -> CAN1_FDC_VMC_MaxAngCtrlOutTqLim/1
  convert_out/1 -> Data Type Conversion/1
  FDCVMCMaxAngCtrlOutTqLim/1 -> convert_out/1

== system halout/HAL_OUT/CAN1/VMC_FCM1_0x172/VMCACCComfortBandLower ==
  VMCACCComfortBandLower : Inport
  Data Type Conversion : DataTypeConversion  OutDataTypeStr=uint16  RndMeth=Round
  convert_out : FVT_lib/hal/convert_out  gain=0.05  offset=-15
  CAN1_VMC_ACC_ComfortBandLower : Outport
  wires:
  Data Type Conversion/1 -> CAN1_VMC_ACC_ComfortBandLower/1
  convert_out/1 -> Data Type Conversion/1
  VMCACCComfortBandLower/1 -> convert_out/1

== system halout/HAL_OUT/CAN1/VMC_FCM1_0x172/VMCACCComfortBandUpper ==
  VMCACCComfortBandUpper : Inport
  Data Type Conversion : DataTypeConversion  OutDataTypeStr=uint16  RndMeth=Round
  convert_out : FVT_lib/hal/convert_out  gain=0.05  offset=-15
  CAN1_VMC_ACC_ComfortBandUpper : Outport
  wires:
  Data Type Conversion/1 -> CAN1_VMC_ACC_ComfortBandUpper/1
  convert_out/1 -> Data Type Conversion/1
  VMCACCComfortBandUpper/1 -> convert_out/1

== system halout/HAL_OUT/CAN1/VMC_FCM1_0x172/VMCACCJerkLowerLInit ==
  VMCACCJerkLowerLInit : Inport
  Data Type Conversion : DataTypeConversion  OutDataTypeStr=uint8  RndMeth=Round
  convert_out : FVT_lib/hal/convert_out  gain=0.1  offset=-6
  CAN1_VMC_ACC_JerkLowerLInit : Outport
  wires:
  Data Type Conversion/1 -> CAN1_VMC_ACC_JerkLowerLInit/1
  convert_out/1 -> Data Type Conversion/1
  VMCACCJerkLowerLInit/1 -> convert_out/1

== system halout/HAL_OUT/CAN1/VMC_FCM1_0x172/VMCACCJerkUpperLInit ==
  VMCACCJerkUpperLInit : Inport
  Data Type Conversion : DataTypeConversion  OutDataTypeStr=uint8  RndMeth=Round
  convert_out : FVT_lib/hal/convert_out  gain=0.1  offset=-6
  CAN1_VMC_ACC_JerkUpperLInit : Outport
  wires:
  Data Type Conversion/1 -> CAN1_VMC_ACC_JerkUpperLInit/1
  convert_out/1 -> Data Type Conversion/1
  VMCACCJerkUpperLInit/1 -> convert_out/1

== system halout/HAL_OUT/CAN1/VMC_FCM1_0x172/VMCACCRequiredAccel ==
  VMCACCRequiredAccel : Inport
  Data Type Conversion : DataTypeConversion  OutDataTypeStr=uint16  RndMeth=Round
  convert_out : FVT_lib/hal/convert_out  gain=0.05  offset=-15
  CAN1_VMC_ACC_RequiredAccel : Outport
  wires:
  Data Type Conversion/1 -> CAN1_VMC_ACC_RequiredAccel/1
  convert_out/1 -> Data Type Conversion/1
  VMCACCRequiredAccel/1 -> convert_out/1

== system halout/HAL_OUT/CAN1/VMC_FCM1_0x172/VMCACCVehHoldReq ==
  VMCACCVehHoldReq : Inport
  Data Type Conversion : DataTypeConversion  OutDataTypeStr=uint8  RndMeth=Round
  CAN1_VMC_ACC_VehHoldReq : Outport
  wires:
  Data Type Conversion/1 -> CAN1_VMC_ACC_VehHoldReq/1
  VMCACCVehHoldReq/1 -> Data Type Conversion/1

== system halout/HAL_OUT/CAN1/VMC_FCM1_0x172/VMCADASACCSta ==
  VMCADASACCSta : Inport
  Data Type Conversion : DataTypeConversion  OutDataTypeStr=uint8  RndMeth=Round
  CAN1_VMC_ADAS_ACC_Sta : Outport
  wires:
  Data Type Conversion/1 -> CAN1_VMC_ADAS_ACC_Sta/1
  VMCADASACCSta/1 -> Data Type Conversion/1

== system halout/HAL_OUT/CAN1/VMC_FCM1_0x172/VMCADASAEBReq ==
  VMCADASAEBReq : Inport
  Data Type Conversion : DataTypeConversion  OutDataTypeStr=uint8  RndMeth=Round
  CAN1_VMC_ADAS_AEBReq : Outport
  wires:
  Data Type Conversion/1 -> CAN1_VMC_ADAS_AEBReq/1
  VMCADASAEBReq/1 -> Data Type Conversion/1

== system halout/HAL_OUT/CAN1/VMC_FCM1_0x172/VMCADASAEBSta ==
  VMCADASAEBSta : Inport
  Data Type Conversion : DataTypeConversion  OutDataTypeStr=uint8  RndMeth=Round
  CAN1_VMC_ADAS_AEB_Sta : Outport
  wires:
  Data Type Conversion/1 -> CAN1_VMC_ADAS_AEB_Sta/1
  VMCADASAEBSta/1 -> Data Type Conversion/1

== system halout/HAL_OUT/CAN1/VMC_FCM1_0x172/VMCADASDBSReq ==
  VMCADASDBSReq : Inport
  Data Type Conversion : DataTypeConversion  OutDataTypeStr=uint8  RndMeth=Round
  CAN1_VMC_ADAS_DBSReq : Outport
  wires:
  Data Type Conversion/1 -> CAN1_VMC_ADAS_DBSReq/1
  VMCADASDBSReq/1 -> Data Type Conversion/1

== system halout/HAL_OUT/CAN1/VMC_FCM1_0x172/VMCADASFaultSta ==
  VMCADASFaultSta : Inport
  Data Type Conversion : DataTypeConversion  OutDataTypeStr=uint8  RndMeth=Round
  CAN1_VMC_ADAS_FaultSta : Outport
  wires:
  Data Type Conversion/1 -> CAN1_VMC_ADAS_FaultSta/1
  VMCADASFaultSta/1 -> Data Type Conversion/1

== system halout/HAL_OUT/CAN1/VMC_FCM1_0x172/VMCAEBVehHoldReq ==
  VMCAEBVehHoldReq : Inport
  Data Type Conversion : DataTypeConversion  OutDataTypeStr=uint8  RndMeth=Round
  CAN1_VMC_AEB_VehHoldReq : Outport
  wires:
  Data Type Conversion/1 -> CAN1_VMC_AEB_VehHoldReq/1
  VMCAEBVehHoldReq/1 -> Data Type Conversion/1

== system halout/HAL_OUT/CAN1/VMC_FCM1_0x172/VMCFCM1Checksum ==
  VMCFCM1Checksum : Inport
  Data Type Conversion : DataTypeConversion  OutDataTypeStr=uint8  RndMeth=Round
  CAN1_VMC_FCM1_Checksum : Outport
  wires:
  Data Type Conversion/1 -> CAN1_VMC_FCM1_Checksum/1
  VMCFCM1Checksum/1 -> Data Type Conversion/1

== system halout/HAL_OUT/CAN1/VMC_FCM1_0x172/VMCFCM1LifeCount ==
  VMCFCM1LifeCount : Inport
  Data Type Conversion : DataTypeConversion  OutDataTypeStr=uint8  RndMeth=Round
  CAN1_VMC_FCM1_LifeCount : Outport
  wires:
  Data Type Conversion/1 -> CAN1_VMC_FCM1_LifeCount/1
  VMCFCM1LifeCount/1 -> Data Type Conversion/1

== system halout/HAL_OUT/CAN1/VMC_FCM1_0x172/VMCFCMLDWFault ==
  VMCFCMLDWFault : Inport
  Data Type Conversion : DataTypeConversion  OutDataTypeStr=uint8  RndMeth=Round
  CAN1_VMC_FCM_LDW_Fault : Outport
  wires:
  Data Type Conversion/1 -> CAN1_VMC_FCM_LDW_Fault/1
  VMCFCMLDWFault/1 -> Data Type Conversion/1

== system halout/HAL_OUT/CAN1/VMC_FCM1_0x172/VMCFCMLDWRequest ==
  VMCFCMLDWRequest : Inport
  Data Type Conversion : DataTypeConversion  OutDataTypeStr=uint8  RndMeth=Round
  CAN1_VMC_FCM_LDW_Request : Outport
  wires:
  Data Type Conversion/1 -> CAN1_VMC_FCM_LDW_Request/1
  VMCFCMLDWRequest/1 -> Data Type Conversion/1

== system halout/HAL_OUT/CAN1/VMC_FCM1_0x172/VMCFCMLKAStrToqReq ==
  VMCFCMLKAStrToqReq : Inport
  Data Type Conversion : DataTypeConversion  OutDataTypeStr=uint16  RndMeth=Round
  convert_out : FVT_lib/hal/convert_out  gain=0.008  offset=-8
  CAN1_VMC_FCM_LKA_StrToqReq : Outport
  wires:
  Data Type Conversion/1 -> CAN1_VMC_FCM_LKA_StrToqReq/1
  convert_out/1 -> Data Type Conversion/1
  VMCFCMLKAStrToqReq/1 -> convert_out/1

== system halout/HAL_OUT/CAN1/VMC_FCM1_0x172/VMCFCMLKATOIAct ==
  VMCFCMLKATOIAct : Inport
  Data Type Conversion : DataTypeConversion  OutDataTypeStr=uint8  RndMeth=Round
  CAN1_VMC_FCM_LKA_TOIAct : Outport
  wires:
  Data Type Conversion/1 -> CAN1_VMC_FCM_LKA_TOIAct/1
  VMCFCMLKATOIAct/1 -> Data Type Conversion/1

== system halout/HAL_OUT/CAN1/VMC_FCM1_0x172/VMCFCMLKATOIFault ==
  VMCFCMLKATOIFault : Inport
  Data Type Conversion : DataTypeConversion  OutDataTypeStr=uint8  RndMeth=Round
  CAN1_VMC_FCM_LKA_TOIFault : Outport
  wires:
  Data Type Conversion/1 -> CAN1_VMC_FCM_LKA_TOIFault/1
  VMCFCMLKATOIFault/1 -> Data Type Conversion/1

== system halout/HAL_OUT/CAN2/FD2_C20_0_0x210/APSExitCondition ==
  APSExitCondition : Inport
  Data Type Conversion : DataTypeConversion  OutDataTypeStr=uint8  RndMeth=Round
  CAN2_APS_ExitCondition : Outport
  wires:
  Data Type Conversion/1 -> CAN2_APS_ExitCondition/1
  APSExitCondition/1 -> Data Type Conversion/1

== system halout/HAL_OUT/CAN2/FD2_C20_0_0x210/APSRQDisplay ==
  APSRQDisplay : Inport
  Data Type Conversion : DataTypeConversion  OutDataTypeStr=uint8  RndMeth=Round
  CAN2_APS_RQ_Display : Outport
  wires:
  Data Type Conversion/1 -> CAN2_APS_RQ_Display/1
  APSRQDisplay/1 -> Data Type Conversion/1

== system halout/HAL_OUT/CAN2/FD2_C20_0_0x210/APSSWVer ==
  APSSWVer : Inport
  Data Type Conversion : DataTypeConversion  OutDataTypeStr=uint8  RndMeth=Round
  CAN2_APS_SW_Ver : Outport
  wires:
  Data Type Conversion/1 -> CAN2_APS_SW_Ver/1
  APSSWVer/1 -> Data Type Conversion/1

== system halout/HAL_OUT/CAN2/FD2_C20_0_0x210/APSStaSystem ==
  APSStaSystem : Inport
  Data Type Conversion : DataTypeConversion  OutDataTypeStr=uint8  RndMeth=Round
  CAN2_APS_Sta_System : Outport
  wires:
  Data Type Conversion/1 -> CAN2_APS_Sta_System/1
  APSStaSystem/1 -> Data Type Conversion/1

== system halout/HAL_OUT/CAN2/FD2_C20_0_0x210/CAASSta ==
  CAASSta : Inport
  Data Type Conversion : DataTypeConversion  OutDataTypeStr=uint8  RndMeth=Round
  CAN2_CAAS_Sta : Outport
  wires:
  Data Type Conversion/1 -> CAN2_CAAS_Sta/1
  CAASSta/1 -> Data Type Conversion/1

== system halout/HAL_OUT/CAN2/FD2_C20_0_0x210/DISCDISCTargetSpd ==
  DISCDISCTargetSpd : Inport
  Data Type Conversion : DataTypeConversion  OutDataTypeStr=uint16  RndMeth=Round
  convert_out : FVT_lib/hal/convert_out  gain=0.125  offset=0
  CAN2_DISC_DISCTargetSpd : Outport
  wires:
  Data Type Conversion/1 -> CAN2_DISC_DISCTargetSpd/1
  convert_out/1 -> Data Type Conversion/1
  DISCDISCTargetSpd/1 -> convert_out/1

== system halout/HAL_OUT/CAN2/FD2_C20_0_0x210/FDCVCURegenLimIndSta ==
  FDCVCURegenLimIndSta : Inport
  Data Type Conversion : DataTypeConversion  OutDataTypeStr=uint8  RndMeth=Round
  CAN2_FDC_VCU_RegenLimInd_Sta : Outport
  wires:
  Data Type Conversion/1 -> CAN2_FDC_VCU_RegenLimInd_Sta/1
  FDCVCURegenLimIndSta/1 -> Data Type Conversion/1

== system halout/HAL_OUT/CAN2/FD2_C20_0_0x210/FDCVCURegenModeSta ==
  FDCVCURegenModeSta : Inport
  Data Type Conversion : DataTypeConversion  OutDataTypeStr=uint8  RndMeth=Round
  CAN2_FDC_VCU_RegenMode_Sta : Outport
  wires:
  Data Type Conversion/1 -> CAN2_FDC_VCU_RegenMode_Sta/1
  FDCVCURegenModeSta/1 -> Data Type Conversion/1

== system halout/HAL_OUT/CAN2/FD2_C20_0_0x210/FDCVCUSimSoundCmd ==
  FDCVCUSimSoundCmd : Inport
  Data Type Conversion : DataTypeConversion  OutDataTypeStr=uint16  RndMeth=Round
  convert_out : FVT_lib/hal/convert_out  gain=0.1  offset=-204.7
  CAN2_FDC_VCU_SimSound_Cmd : Outport
  wires:
  Data Type Conversion/1 -> CAN2_FDC_VCU_SimSound_Cmd/1
  convert_out/1 -> Data Type Conversion/1
  FDCVCUSimSoundCmd/1 -> convert_out/1

== system halout/HAL_OUT/CAN2/FD2_C20_0_0x210/FDCVCUSmartEcoSpdLimSta ==
  FDCVCUSmartEcoSpdLimSta : Inport
  Data Type Conversion : DataTypeConversion  OutDataTypeStr=uint8  RndMeth=Round
  CAN2_FDC_VCU_SmartEcoSpdLim_Sta : Outport
  wires:
  Data Type Conversion/1 -> CAN2_FDC_VCU_SmartEcoSpdLim_Sta/1
  FDCVCUSmartEcoSpdLimSta/1 -> Data Type Conversion/1

== system halout/HAL_OUT/CAN2/FD2_C20_0_0x210/FDCVCUSmartEcoSta ==
  FDCVCUSmartEcoSta : Inport
  Data Type Conversion : DataTypeConversion  OutDataTypeStr=uint8  RndMeth=Round
  CAN2_FDC_VCU_SmartEco_Sta : Outport
  wires:
  Data Type Conversion/1 -> CAN2_FDC_VCU_SmartEco_Sta/1
  FDCVCUSmartEcoSta/1 -> Data Type Conversion/1

== system halout/HAL_OUT/CAN2/FD2_C20_0_0x210/FDCVMCSetSpdDispSta ==
  FDCVMCSetSpdDispSta : Inport
  Data Type Conversion : DataTypeConversion  OutDataTypeStr=uint8  RndMeth=Round
  CAN2_FDC_VMC_SetSpdDisp_Sta : Outport
  wires:
  Data Type Conversion/1 -> CAN2_FDC_VMC_SetSpdDisp_Sta/1
  FDCVMCSetSpdDispSta/1 -> Data Type Conversion/1

== system halout/HAL_OUT/CAN2/FD2_C20_0_0x210/FDCVMCSetSpdSta ==
  FDCVMCSetSpdSta : Inport
  Data Type Conversion : DataTypeConversion  OutDataTypeStr=uint8  RndMeth=Round
  CAN2_FDC_VMC_SetSpd_Sta : Outport
  wires:
  Data Type Conversion/1 -> CAN2_FDC_VMC_SetSpd_Sta/1
  FDCVMCSetSpdSta/1 -> Data Type Conversion/1

== system halout/HAL_OUT/CAN2/FD2_C20_0_0x210/FDCVMCSpdCtrlModeSta ==
  FDCVMCSpdCtrlModeSta : Inport
  Data Type Conversion : DataTypeConversion  OutDataTypeStr=uint8  RndMeth=Round
  CAN2_FDC_VMC_SpdCtrlMode_Sta : Outport
  wires:
  Data Type Conversion/1 -> CAN2_FDC_VMC_SpdCtrlMode_Sta/1
  FDCVMCSpdCtrlModeSta/1 -> Data Type Conversion/1

== system halout/HAL_OUT/CAN2/FD2_C20_0_0x210/FDCVMCSpdCtrlSta ==
  FDCVMCSpdCtrlSta : Inport
  Data Type Conversion : DataTypeConversion  OutDataTypeStr=uint8  RndMeth=Round
  CAN2_FDC_VMC_SpdCtrl_Sta : Outport
  wires:
  Data Type Conversion/1 -> CAN2_FDC_VMC_SpdCtrl_Sta/1
  FDCVMCSpdCtrlSta/1 -> Data Type Conversion/1

== system halout/HAL_OUT/CAN2/FD2_C20_0_0x210/PASAFCL ==
  PASAFCL : Inport
  Data Type Conversion : DataTypeConversion  OutDataTypeStr=uint8  RndMeth=Round
  CAN2_PAS_A_FCL : Outport
  wires:
  Data Type Conversion/1 -> CAN2_PAS_A_FCL/1
  PASAFCL/1 -> Data Type Conversion/1

== system halout/HAL_OUT/CAN2/FD2_C20_0_0x210/PASAFCR ==
  PASAFCR : Inport
  Data Type Conversion : DataTypeConversion  OutDataTypeStr=uint8  RndMeth=Round
  CAN2_PAS_A_FCR : Outport
  wires:
  Data Type Conversion/1 -> CAN2_PAS_A_FCR/1
  PASAFCR/1 -> Data Type Conversion/1

== system halout/HAL_OUT/CAN2/FD2_C20_0_0x210/PASAFML ==
  PASAFML : Inport
  Data Type Conversion : DataTypeConversion  OutDataTypeStr=uint8  RndMeth=Round
  CAN2_PAS_A_FML : Outport
  wires:
  Data Type Conversion/1 -> CAN2_PAS_A_FML/1
  PASAFML/1 -> Data Type Conversion/1

== system halout/HAL_OUT/CAN2/FD2_C20_0_0x210/PASAFMR ==
  PASAFMR : Inport
  Data Type Conversion : DataTypeConversion  OutDataTypeStr=uint8  RndMeth=Round
  CAN2_PAS_A_FMR : Outport
  wires:
  Data Type Conversion/1 -> CAN2_PAS_A_FMR/1
  PASAFMR/1 -> Data Type Conversion/1

== system halout/HAL_OUT/CAN2/FD2_C20_0_0x210/PASARCL ==
  PASARCL : Inport
  Data Type Conversion : DataTypeConversion  OutDataTypeStr=uint8  RndMeth=Round
  CAN2_PAS_A_RCL : Outport
  wires:
  Data Type Conversion/1 -> CAN2_PAS_A_RCL/1
  PASARCL/1 -> Data Type Conversion/1

== system halout/HAL_OUT/CAN2/FD2_C20_0_0x210/PASARCR ==
  PASARCR : Inport
  Data Type Conversion : DataTypeConversion  OutDataTypeStr=uint8  RndMeth=Round
  CAN2_PAS_A_RCR : Outport
  wires:
  Data Type Conversion/1 -> CAN2_PAS_A_RCR/1
  PASARCR/1 -> Data Type Conversion/1

== system halout/HAL_OUT/CAN2/FD2_C20_0_0x210/PASARML ==
  PASARML : Inport
  Data Type Conversion : DataTypeConversion  OutDataTypeStr=uint8  RndMeth=Round
  CAN2_PAS_A_RML : Outport
  wires:
  Data Type Conversion/1 -> CAN2_PAS_A_RML/1
  PASARML/1 -> Data Type Conversion/1

== system halout/HAL_OUT/CAN2/FD2_C20_0_0x210/PASARMR ==
  PASARMR : Inport
  Data Type Conversion : DataTypeConversion  OutDataTypeStr=uint8  RndMeth=Round
  CAN2_PAS_A_RMR : Outport
  wires:
  Data Type Conversion/1 -> CAN2_PAS_A_RMR/1
  PASARMR/1 -> Data Type Conversion/1

== system halout/HAL_OUT/CAN2/FD2_C20_0_0x210/PASChime ==
  PASChime : Inport
  Data Type Conversion : DataTypeConversion  OutDataTypeStr=uint8  RndMeth=Round
  CAN2_PAS_Chime : Outport
  wires:
  Data Type Conversion/1 -> CAN2_PAS_Chime/1
  PASChime/1 -> Data Type Conversion/1

== system halout/HAL_OUT/CAN2/FD2_C20_0_0x210/PASDFCL ==
  PASDFCL : Inport
  Data Type Conversion : DataTypeConversion  OutDataTypeStr=uint8  RndMeth=Round
  CAN2_PAS_D_FCL : Outport
  wires:
  Data Type Conversion/1 -> CAN2_PAS_D_FCL/1
  PASDFCL/1 -> Data Type Conversion/1

== system halout/HAL_OUT/CAN2/FD2_C20_0_0x210/PASDFCR ==
  PASDFCR : Inport
  Data Type Conversion : DataTypeConversion  OutDataTypeStr=uint8  RndMeth=Round
  CAN2_PAS_D_FCR : Outport
  wires:
  Data Type Conversion/1 -> CAN2_PAS_D_FCR/1
  PASDFCR/1 -> Data Type Conversion/1

== system halout/HAL_OUT/CAN2/FD2_C20_0_0x210/PASDFML ==
  PASDFML : Inport
  Data Type Conversion : DataTypeConversion  OutDataTypeStr=uint8  RndMeth=Round
  CAN2_PAS_D_FML : Outport
  wires:
  Data Type Conversion/1 -> CAN2_PAS_D_FML/1
  PASDFML/1 -> Data Type Conversion/1

== system halout/HAL_OUT/CAN2/FD2_C20_0_0x210/PASDFMR ==
  PASDFMR : Inport
  Data Type Conversion : DataTypeConversion  OutDataTypeStr=uint8  RndMeth=Round
  CAN2_PAS_D_FMR : Outport
  wires:
  Data Type Conversion/1 -> CAN2_PAS_D_FMR/1
  PASDFMR/1 -> Data Type Conversion/1

== system halout/HAL_OUT/CAN2/FD2_C20_0_0x210/PASDRCL ==
  PASDRCL : Inport
  Data Type Conversion : DataTypeConversion  OutDataTypeStr=uint8  RndMeth=Round
  CAN2_PAS_D_RCL : Outport
  wires:
  Data Type Conversion/1 -> CAN2_PAS_D_RCL/1
  PASDRCL/1 -> Data Type Conversion/1
